simulink model "hishlevelSintes"  (R2023a)
settings: Solver=VariableStepAuto  StartTime=0.0  StopTime=10.0  RelTol=1e-3
settings Model: Creator=mehra  LastModifiedBy=mehra

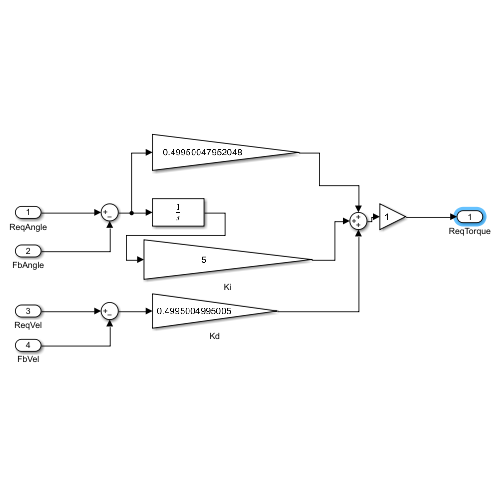
[thumbnail: Simulink's stored preview of the top-level diagram]
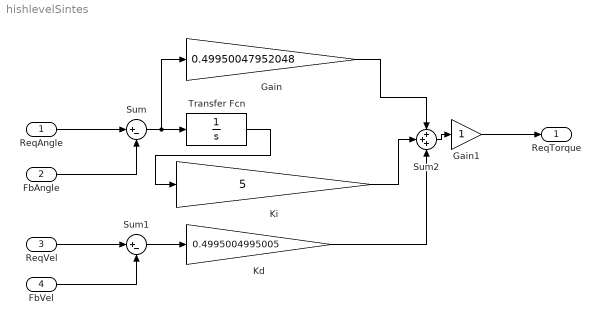
== system hishlevelSintes ==
  ReqAngle : Inport
  FbAngle : Inport  Port=2
  ReqVel : Inport  Port=3
  FbVel : Inport  Port=4
  Gain : Gain  Gain=0.49950047952048
  Gain1 : Gain
  Kd : Gain  Gain=0.4995004995005
  Ki : Gain  Gain=5
  Sum : Sum  Inputs=|+-
  Sum1 : Sum  Inputs=|+-
  Sum2 : Sum  Inputs=+++
  Transfer Fcn : TransferFcn  Denominator=[1 0]
  ReqTorque : Outport
  wires:
  Sum/1 -> Transfer Fcn/1, Gain/1
  Sum2/1 -> Gain1/1
  Sum1/1 -> Kd/1
  ReqAngle/1 -> Sum/1
  Gain/1 -> Sum2/1
  Kd/1 -> Sum2/3
  Transfer Fcn/1 -> Ki/1
  FbVel/1 -> Sum1/2
  ReqVel/1 -> Sum1/1
  FbAngle/1 -> Sum/2
  Ki/1 -> Sum2/2
  Gain1/1 -> ReqTorque/1
